simulink model "part2_LQR1_sim"  (R2017a)
settings: Solver=VariableStepAuto  StartTime=0.0  StopTime=simTime  RelTol=1e-3
values from neighbouring files (symbols this model uses):
  A = [0 0 0 0 0 0 40.7055790872 38.6368253303 1 0 -13.2363115295 -4.71950452077 ... (16 elements, 4x4)]    [model.mat]    (also in part1_lin_model.m = [)
  B = [0 0 23.29957643 8.30763585823]    [model.mat]    (also in part1_lin_model.m = [)
  C = [1  0  0  0; 0  1  0  0]    [model.mat]    (also in part1_lin_model.m = eye(2,4))
  D = [0 0]    [model.mat]    (also in part1_lin_model.m = zeros(2,1))
  power_noise = 1*10^-8    (= 1e-08)    [part2_designController.m]    (also in part3_designController.m = 0; part4.m = 0)
  simTime = 10    [part2_designController.m]    (also in part3_designController.m)
  theta_d = 1    [part2_designController.m]    (also in part3_designController.m; part4.m)
  Ts = 1/200    (= 0.005)    [part2_designController.m]    (also in part3_designController.m; part4.m)
  x0 = [0;0;0;0]    [part2_designController.m]    (also in part3_designController.m; part4.m)
undefined symbols (not defined in the file or in its folder): K
libraries: simulink x1
settings Model: Creator=zilleplus  LastModifiedBy=Maarten

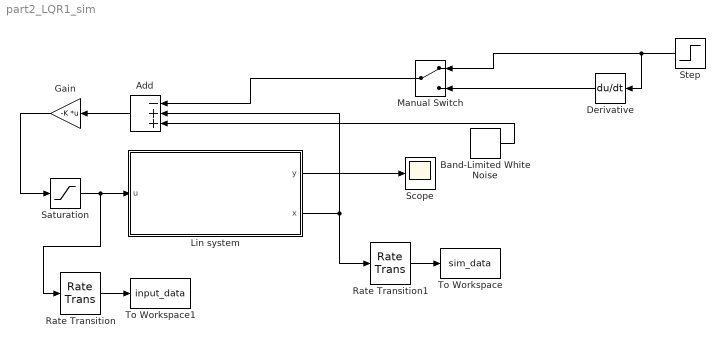
== system part2_LQR1_sim ==
  Add : Sum  Inputs=-++
  Band-Limited White Noise : simulink/Sources/Band-Limited White Noise  Cov=power_noise*ones(4,1)  Ts=Ts  seed=[23341]
  Derivative : Derivative  CoefficientInTFapproximation=1
  Gain : Gain  Gain=-K  Multiplication=Matrix(K*u) (u vector)
  Lin system : Subsystem
  Manual Switch : ManualSwitch
  Rate Transition : RateTransition
  Rate Transition1 : RateTransition  OutPortSampleTime=Ts
  Saturation : Saturate  UpperLimit=5  LowerLimit=-5
  Scope : Scope
  Step : Step  Time=0.1*simTime  Before=x0  After=[theta_d;0;0;0]  SampleTime=0
  To Workspace : ToWorkspace  VariableName=sim_data  SaveFormat=Timeseries  SampleTime=-1
  To Workspace1 : ToWorkspace  VariableName=input_data  SaveFormat=Timeseries  SampleTime=Ts
  wires:
  Gain/1 -> Saturation/1
  Lin system/1(y) -> Scope/1
  Lin system/2(x) -> Rate Transition1/1, Add/2
  Add/1 -> Gain/1
  Saturation/1 -> Rate Transition/1, Lin system/1(u)
  Rate Transition/1 -> To Workspace1/1
  Rate Transition1/1 -> To Workspace/1
  Band-Limited White Noise/1 -> Add/3
  Step/1 -> Manual Switch/1, Derivative/1
  Manual Switch/1 -> Add/1
  Derivative/1 -> Manual Switch/2

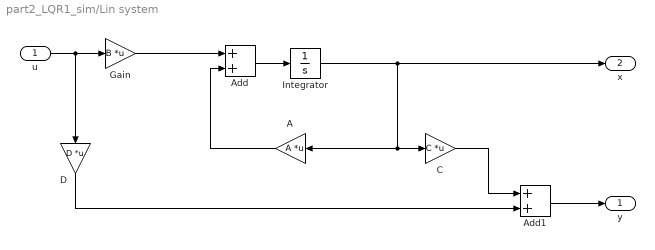
== system part2_LQR1_sim/Lin system ==
  u : Inport
  A : Gain  Gain=A  Multiplication=Matrix(K*u) (u vector)
  Add : Sum
  Add1 : Sum
  C : Gain  Gain=C  Multiplication=Matrix(K*u) (u vector)
  D : Gain  Gain=D  Multiplication=Matrix(K*u) (u vector)
  Gain : Gain  Gain=B  Multiplication=Matrix(K*u) (u vector)
  Integrator : Integrator  InitialCondition=x0
  y : Outport
  x : Outport  Port=2
  wires:
  u/1 -> D/1, Gain/1
  Integrator/1 -> x/1, A/1, C/1
  A/1 -> Add/2
  Gain/1 -> Add/1
  C/1 -> Add1/1
  Add1/1 -> y/1
  D/1 -> Add1/2
  Add/1 -> Integrator/1
